simulink model "kinematic_on_real_system"  (R2016b)
settings: Solver=FixedStepAuto  StartTime=0.0  StopTime=100  FixedStep=0.04  RelTol=1e-3  EnableMultiTasking=on
values from neighbouring files (symbols this model uses):
  Cx = [0 0 1 0 0 0;0 0 0 1 0 0;0 0 0 0 1 0; 0 0 0 0 0 1]    [lqgfin.m]
  Cy = [1 0 0 0 0 0;0 1 0 0 0 0]    [lqgfin.m]
  l = 0.21    [lqgfin.m]
  ly = 0.1    [lqgfin.m]
  r = 0.13/2    (= 0.065)    [lqgfin.m]
  u_51 = [[-5:0.2:-3],[-2.9:0.1:2.9],[3:0.2:5]]    [lqgfin.m]
  vol_l = [-[10.3,9.95,9.86,9.8,9.74,9.65,9.53,9.42,9.3,9.15,8.98,8.86,     8.75,8.64,8.53,8.39,8.25,8.05,7.9,7.6,7.4,7.1,6.88,6.48,6.1,5.7,     5.2,4.7,4.13,3.45,2.7,1.75,0.21,0.165,0.12,0.088,0.06,0.036,0.017,     0.005],[0,0.005,0.017,0.035,0.061,0.092,0.122,0.160,0.960,1.7,2.6,     3.25,4,4.6,5.1,5.6,6,6.44,6.8,7.1,7.4,7.65,7.8,8,8.11,8.25,8.4,     8.55,8.68,8.82,8.95,9.15,9.29,9.44,9.56,9.67,9.75,9.82, ...(+23 chars)    [lqgfin.m]
  vol_r = [-[10.31,9.98,9.88,9.8,9.72,9.62,9.5,9.37,9.22,9.05,8.87,8.73,     8.62,8.49,8.35,8.19,8.01,7.84,7.63,7.41,7.16,6.76,6.43,6.09,5.68,     5.22,4.74,4.16,3.56,2.92,2.15,0.42,0.35,0.032,0.027,0.023,0.019,     0.013,0.0068,0.00156],[0,0.0013,0.0018,0.006,0.012,0.018,0.026,     0.032,0.109,1.16,2,2.67,3.35,4.05,4.61,5.12,5.59,6.00,6.35,6.69,     7.06,7.29,7.55,7.77,7.96,8.14,8.31,8.45,8.59,8.72,8.86,9. ...(+55 chars)    [lqgfin.m]
undefined symbols (not defined in the file or in its folder): An, Bn, Cn, codertarget, Dn, gcbh, K_lqi
libraries: simulink x9, arduinolib x4, Controllers x2, MinSegLibrary_M1V4 x2, DiffSteer_model x1
settings Model: SimulationMode=external  ExtModeTrigDuration=2  Creator=Hamza  LastModifiedBy=Hamza
settings OptimizationCC: MaxStackSize=64
settings DebuggingCC: ParameterTunabilityLossMsg=error
settings HardwareCC: ProdBitPerPointer=32  ProdBitPerSizeT=32  ProdBitPerPtrDiffT=32  ProdLargestAtomicInteger=Long  ProdLargestAtomicFloat=Double  ProdWordSize=32  ProdHWDeviceType=ARM Compatible->ARM Cortex
settings RTWCC: SystemTargetFile=ert.tlc  HardwareBoard=Arduino Due  TLCOptions=-aInlineSetEventsForThisBaseRateFcn=TLC_FALSE -aSuppressMultiTaskScheduler=TLC_FALSE -aRateBasedStepFcn=1  TemplateMakefile=ert_default_tmf  Description=Embedded Coder  GenerateReport=on  Toolchain=Arduino ARM  BuildConfiguration=Faster Runs  IncludeHyperlinkInReport=on  LaunchReport=on  GenerateTraceInfo=on  GenerateTraceReport=on  GenerateTraceReportSl=on  GenerateTraceReportSf=on  GenerateTraceReportEml=on
settings CodeAppCC: ForceParamTrailComments=on  IgnoreCustomStorageClasses=off  OperatorAnnotations=on  SimulinkDataObjDesc=on  SFDataObjDesc=on  MATLABFcnDesc=on  InsertBlockDesc=on  MATLABSourceComments=on
settings ERTTargetCC: SupportContinuousTime=on  SupportVariableSizeSignals=on  ExtMode=on  ExtModeMexArgs='127.0.0.1' 0 17725

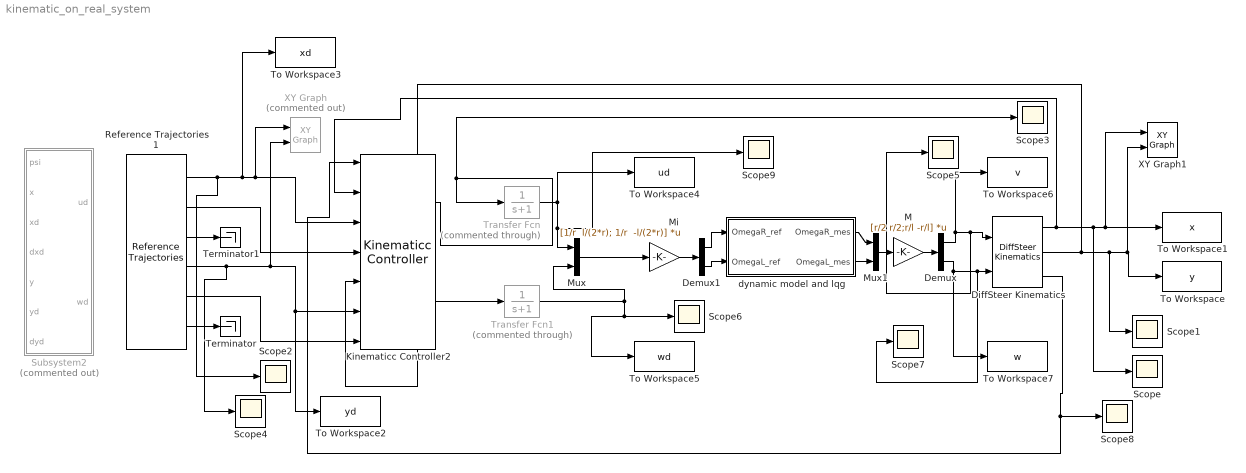
== system kinematic_on_real_system ==
  Demux : Demux  Outputs=2
  Demux1 : Demux  Outputs=2
  DiffSteer Kinematics : DiffSteer_model/DiffSteer Kinematics  x0=[0, 0, 0]  a=0.18  umax=1.3  wmax=12  dumax=5  dwmax=5
  Kinematicc Controller2 : Controllers/Kinematicc Controller  kx=1  ky=1  lx=0.25  ly=0.25  a=0
      link override 1//a: Gain=1/0.18
  M : Gain  Gain=[r/2 r/2;r/l -r/l]  Multiplication=Matrix(K*u)
  Mi : Gain  Gain="[1/r  l/(2*r); 1/r  -l/(2*r)]"  Multiplication=Matrix(K*u)
  Mux : Mux  Inputs=2
  Mux1 : Mux  Inputs=2
  Reference Trajectories1 : Controllers/Reference Trajectories  trajectory_type=1  wf=0.2  raio_ref_1=1.15  delta_raio=-0.1  t_delta_raio=100  xd=[2.5, 2.5]
      link override ganho: Gain=1
      link override zero2: Value=1
  Scope{,1..9} (10 alike) : Scope
  Subsystem2 : Subsystem  Commented=on
  Terminator : Terminator
  Terminator1 : Terminator
  To Workspace : ToWorkspace  VariableName=y  SampleTime=-1
  To Workspace1 : ToWorkspace  VariableName=x  SampleTime=-1
  To Workspace2 : ToWorkspace  VariableName=yd  SampleTime=-1
  To Workspace3 : ToWorkspace  VariableName=xd  SampleTime=-1
  To Workspace4 : ToWorkspace  VariableName=ud  SampleTime=-1
  To Workspace5 : ToWorkspace  VariableName=wd  SampleTime=-1
  To Workspace6 : ToWorkspace  VariableName=v  SampleTime=-1
  To Workspace7 : ToWorkspace  VariableName=w  SampleTime=-1
  Transfer Fcn : TransferFcn  Commented=through  Denominator=[1 1]
  Transfer Fcn1 : TransferFcn  Commented=through  Denominator=[1 1]
  XY Graph : simulink/Sinks/XY Graph  Commented=on  xmin=-2  xmax=50  ymin=-3  ymax=50  st=-1
  XY Graph1 : simulink/Sinks/XY Graph  xmin=-1.5  xmax=1.5  ymin=-1.5  ymax=1.5  st=-1
  dynamic model and lqg : Subsystem
  wires:
  Reference Trajectories1/1 -> Scope2/1, To Workspace3/1, Kinematicc Controller2/3, XY Graph/1
  Reference Trajectories1/2 -> Kinematicc Controller2/4
  Reference Trajectories1/4 -> Scope4/1, XY Graph/2, To Workspace2/1, Kinematicc Controller2/6
  Reference Trajectories1/5 -> Kinematicc Controller2/7
  DiffSteer Kinematics/1 -> Kinematicc Controller2/2, Scope/1, XY Graph1/1, To Workspace1/1
  DiffSteer Kinematics/2 -> Kinematicc Controller2/5, Scope1/1, XY Graph1/2, To Workspace/1
  DiffSteer Kinematics/3 -> Kinematicc Controller2/1, Scope8/1
  Kinematicc Controller2/2 -> Transfer Fcn1/1
  Demux/2 -> Scope7/1, DiffSteer Kinematics/2, To Workspace7/1
  Reference Trajectories1/3 -> Terminator1/1
  Reference Trajectories1/6 -> Terminator/1
  Mux1/1 -> M/1
  Mux/1 -> Mi/1
  M/1 -> Demux/1
  Mi/1 -> Demux1/1
  Demux1/1 -> dynamic model and lqg/1(OmegaR_ref)
  dynamic model and lqg/1(OmegaR_mes) -> Mux1/1
  dynamic model and lqg/2(OmegaL_mes) -> Mux1/2
  Demux/1 -> Scope5/1, DiffSteer Kinematics/1, To Workspace6/1
  Kinematicc Controller2/1 -> Transfer Fcn/1, Scope3/1
  Transfer Fcn/1 -> Scope9/1, Mux/1, To Workspace4/1
  Transfer Fcn1/1 -> To Workspace5/1, Scope6/1, Mux/2
  Demux1/2 -> dynamic model and lqg/2(OmegaL_ref)

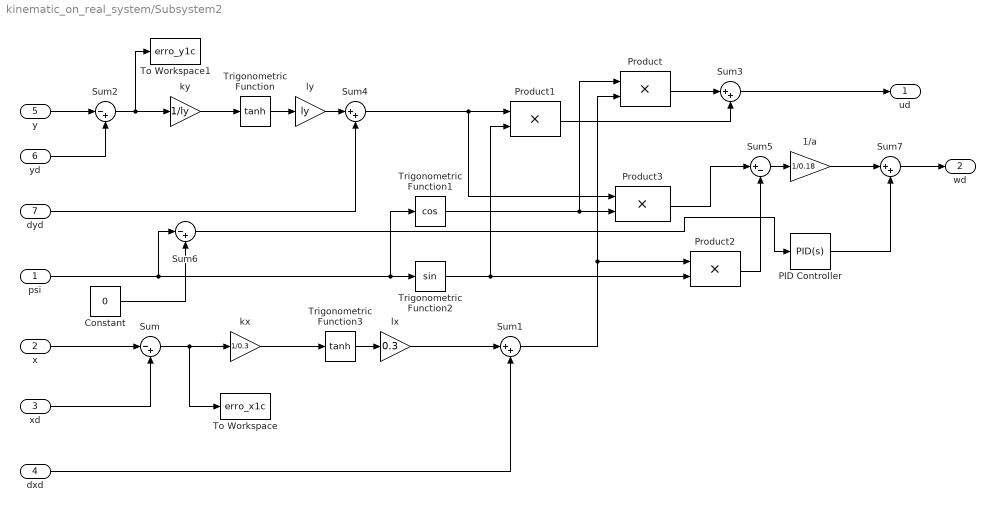
== system kinematic_on_real_system/Subsystem2 ==
  psi : Inport
  x : Inport  Port=2
  xd : Inport  Port=3
  dxd : Inport  Port=4
  y : Inport  Port=5
  yd : Inport  Port=6
  dyd : Inport  Port=7
  1/a : Gain  Gain=1/0.18  SaturateOnIntegerOverflow=on  OutDataTypeStr=Inherit: Same as input  ParamDataTypeStr=Inherit: Same as input
  Constant : Constant  Value=0
  PID Controller : simulink/Continuous/PID Controller  Controller=PID  TimeDomain=Continuous-time  SampleTime=-1  IntegratorMethod=Forward Euler  FilterMethod=Forward Euler  Form=Parallel  UseFilter=on  ControllerParametersSource=internal  P=1  I=0.01  D=0.5  N=100  InitialConditionSource=internal  InitialConditionForIntegrator=0  InitialConditionForFilter=0  ExternalReset=none  LimitOutput=off  UpperSaturationLimit=inf  LowerSaturationLimit=-inf  LinearizeAsGain=on  AntiWindupMode=none  Kb=1  TrackingMode=off  Kt=1  PParamMin=[]  PParamMax=[]  IParamMin=[]  IParamMax=[]  DParamMin=[]  DParamMax=[]  NParamMin=[]  NParamMax=[]  KbParamMin=[]  KbParamMax=[]  KtParamMin=[]  KtParamMax=[]  POutMin=[]  POutMax=[]  IOutMin=[]  IOutMax=[]  DOutMin=[]  DOutMax=[]  NOutMin=[]  NOutMax=[]  KbOutMin=[]  KbOutMax=[]  KtOutMin=[]  KtOutMax=[]  IntegratorOutMin=[]  IntegratorOutMax=[]  FilterOutMin=[]  FilterOutMax=[]  SumOutMin=[]  SumOutMax=[]  SumI1OutMin=[]  SumI1OutMax=[]  SumI2OutMin=[]  SumI2OutMax=[]  SumI3OutMin=[]  SumI3OutMax=[]  SumDOutMin=[]  SumDOutMax=[]  SaturationOutMin=[]  SaturationOutMax=[]  IntegratorContinuousStateAttributes=''  IntegratorStateMustResolveToSignalObject=off  IntegratorRTWStateStorageClass=Auto  FilterContinuousStateAttributes=''  FilterStateMustResolveToSignalObject=off  FilterRTWStateStorageClass=Auto  DifferentiatorICPrevScaledInput=0  DifferentiatorOutMin=[]  DifferentiatorOutMax=[]
  Product{,1..3} (4 alike) : Product  SaturateOnIntegerOverflow=on  OutDataTypeStr=Inherit: Same as first input
  Sum : Sum  Inputs=|-+  SaturateOnIntegerOverflow=on
  Sum{1,3..4,7} (4 alike) : Sum  Inputs=|++  SaturateOnIntegerOverflow=on
  Sum2 : Sum  Inputs=|-+  SaturateOnIntegerOverflow=on
  Sum5 : Sum  Inputs=|+-  SaturateOnIntegerOverflow=on
  Sum6 : Sum  Inputs=|-+  SaturateOnIntegerOverflow=on
  To Workspace : ToWorkspace  VariableName=erro_x1c  SampleTime=-1
  To Workspace1 : ToWorkspace  VariableName=erro_y1c  SampleTime=-1
  Trigonometric Function : Trigonometry  Operator=tanh
  Trigonometric Function1 : Trigonometry  Operator=cos
  Trigonometric Function2 : Trigonometry
  Trigonometric Function3 : Trigonometry  Operator=tanh
  kx : Gain  Gain=1/0.3  SaturateOnIntegerOverflow=on  OutDataTypeStr=Inherit: Same as input  ParamDataTypeStr=Inherit: Same as input
  ky : Gain  Gain=1/ly  SaturateOnIntegerOverflow=on  OutDataTypeStr=Inherit: Same as input  ParamDataTypeStr=Inherit: Same as input
  lx : Gain  Gain=0.3  SaturateOnIntegerOverflow=on  OutDataTypeStr=Inherit: Same as input  ParamDataTypeStr=Inherit: Same as input
  ly : Gain  Gain=ly  SaturateOnIntegerOverflow=on  OutDataTypeStr=Inherit: Same as input  ParamDataTypeStr=Inherit: Same as input
  ud : Outport
  wd : Outport  Port=2
  wires:
  Sum/1 -> kx/1, To Workspace/1
  y/1 -> Sum2/1
  Sum4/1 -> Product1/1, Product3/1
  Trigonometric Function2/1 -> Product2/2, Product1/2
  ky/1 -> Trigonometric Function/1
  kx/1 -> Trigonometric Function3/1
  Trigonometric Function1/1 -> Product3/2, Product/1
  yd/1 -> Sum2/2
  xd/1 -> Sum/2
  x/1 -> Sum/1
  psi/1 -> Sum6/1, Trigonometric Function2/1, Trigonometric Function1/1
  Sum1/1 -> Product2/1, Product/2
  Product1/1 -> Sum3/2
  Product3/1 -> Sum5/1
  Sum2/1 -> ky/1, To Workspace1/1
  Product/1 -> Sum3/1
  Product2/1 -> Sum5/2
  Sum3/1 -> ud/1
  ly/1 -> Sum4/1
  dxd/1 -> Sum1/2
  dyd/1 -> Sum4/2
  Trigonometric Function/1 -> ly/1
  lx/1 -> Sum1/1
  Trigonometric Function3/1 -> lx/1
  Sum7/1 -> wd/1
  Sum5/1 -> 1/a/1
  Sum6/1 -> PID Controller/1
  PID Controller/1 -> Sum7/2
  1/a/1 -> Sum7/1
  Constant/1 -> Sum6/2

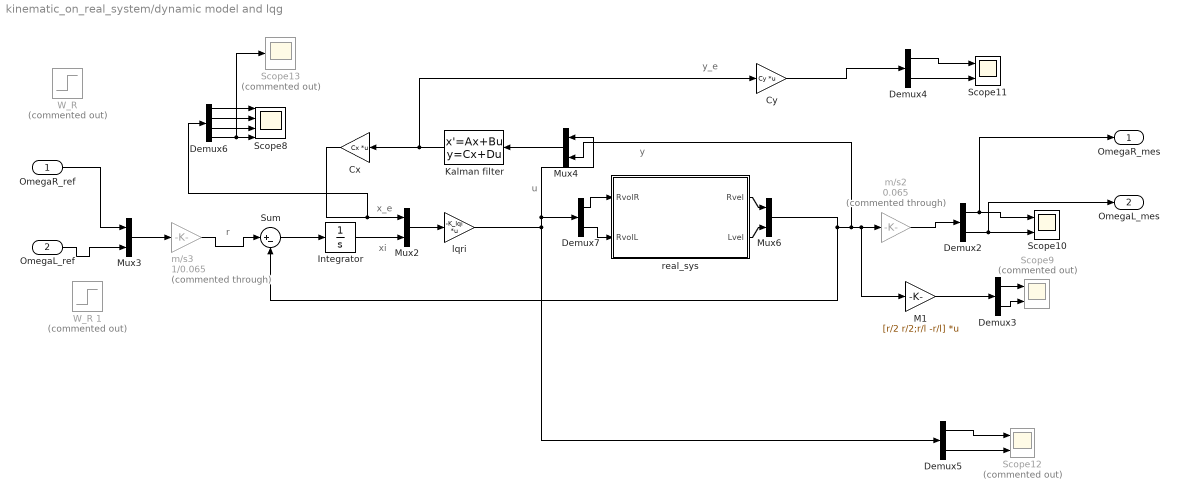
== system kinematic_on_real_system/dynamic model and lqg ==
  note: r
  note: y_e
  note: xi
  note: x_e
  note: u
  note: y
  OmegaR_ref : Inport
  OmegaL_ref : Inport  Port=2
  Cx : Gain  Gain=Cx  Multiplication=Matrix(K*u)
  Cy : Gain  Gain=Cy  Multiplication=Matrix(K*u)
  Demux{2..5,7} (5 alike) : Demux  Outputs=2
  Demux6 : Demux
  Integrator : Integrator
  Kalman filter : StateSpace  A=An  B=Bn  C=Cn  D=Dn  X0=0
  M1 : Gain  Gain=[r/2 r/2;r/l -r/l]  Multiplication=Matrix(K*u)
  Mux{2..4,6} (4 alike) : Mux  Inputs=2
  Scope10 : Scope  NumInputPorts=2
  Scope11 : Scope  NumInputPorts=2
  Scope12 : Scope  Commented=on  NumInputPorts=2
  Scope13 : Scope  Commented=on
  Scope8 : Scope  NumInputPorts=4
  Scope9 : Scope  Commented=on  NumInputPorts=2
  Sum : Sum  Inputs=|+-
  "W_R " : Step  Commented=on  After=10  SampleTime=0.02
  W_R 1 : Step  Commented=on  After=10  SampleTime=0.02
  lqri : Gain  Gain=-K_lqi  Multiplication=Matrix(K*u)
  m/s2 : Gain  Commented=through  Gain=0.065
  m/s3 : Gain  Commented=through  Gain=1/0.065
  "real_sys " : Subsystem
  OmegaR_mes : Outport
  OmegaL_mes : Outport  Port=2
  wires:
  OmegaR_ref/1 -> Mux3/1
  Demux5/1 -> Scope12/1
  Demux7/1 -> "real_sys "/1(RvolR)
  Demux5/2 -> Scope12/2
  "real_sys "/1(Rvel) -> Mux6/1
  Demux7/2 -> "real_sys "/2("RvolL ")
  lqri/1 -> Demux7/1, Mux4/1, Demux5/1
  "real_sys "/2(Lvel) -> Mux6/2
  Demux3/2 -> Scope9/2
  Cx/1 -> Demux6/1, Mux2/1
  M1/1 -> Demux3/1
  Demux6/1 -> Scope8/1
  Mux6/1 -> Sum/2, M1/1, m/s2/1, Mux4/2
  Demux6/2 -> Scope8/2
  Demux6/3 -> Scope8/3
  Demux6/4 -> Scope13/1, Scope8/4
  m/s2/1 -> Demux2/1
  Demux3/1 -> Scope9/1
  m/s3/1 -> Sum/1
  Cy/1 -> Demux4/1
  Sum/1 -> Integrator/1
  Integrator/1 -> Mux2/2
  Mux2/1 -> lqri/1
  Mux3/1 -> m/s3/1
  Demux2/2 -> OmegaL_mes/1, Scope10/2
  Kalman filter/1 -> Cy/1, Cx/1
  Demux4/1 -> Scope11/1
  Mux4/1 -> Kalman filter/1
  OmegaL_ref/1 -> Mux3/2
  Demux2/1 -> OmegaR_mes/1, Scope10/1
  Demux4/2 -> Scope11/2

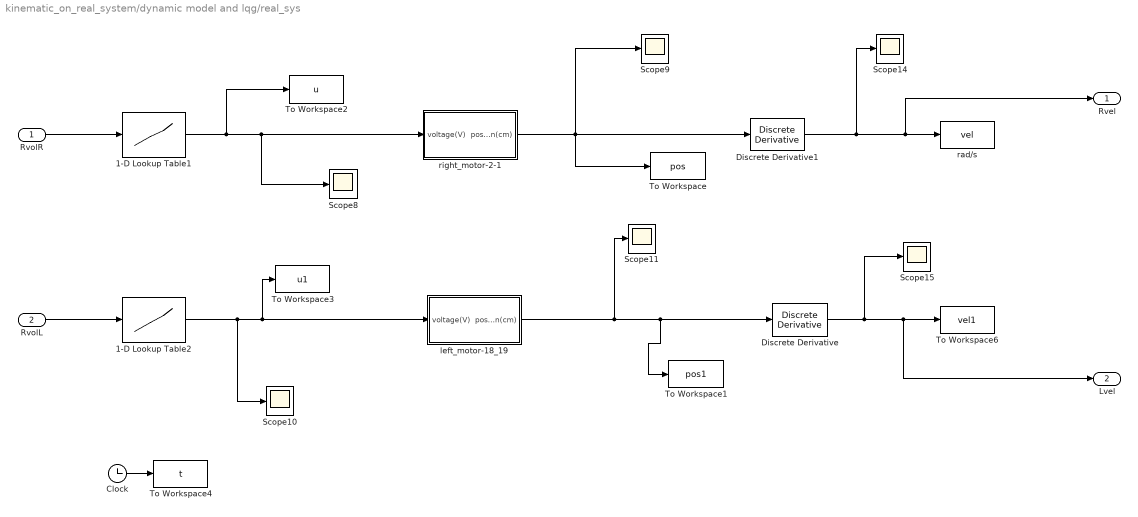
== system kinematic_on_real_system/dynamic model and lqg/real_sys  ==
  RvolR : Inport
  "RvolL " : Inport  Port=2
  1-D Lookup Table1 : Lookup_n-D  NumberOfTableDimensions=1  BreakpointsForDimension1=vol_r  Table=u_51  InternalRulePriority=Speed  RndMeth=Simplest  InputSameDT=on
  1-D Lookup Table2 : Lookup_n-D  NumberOfTableDimensions=1  BreakpointsForDimension1=vol_l  Table=u_51  InternalRulePriority=Speed  RndMeth=Simplest  InputSameDT=on
  Clock : Clock
  Discrete Derivative : simulink/Discrete/Discrete Derivative  gainval=1.0  ICPrevScaledInput=0.0  OutMin=[]  OutMax=[]  OutDataType=fixdt(1, 16)  OutScaling=2^-10  DoSatur=off
  Discrete Derivative1 : simulink/Discrete/Discrete Derivative  gainval=1.0  ICPrevScaledInput=0.0  OutMin=[]  OutMax=[]  OutDataType=fixdt(1, 16)  OutScaling=2^-10  DoSatur=off
  Scope{8..11,14..15} (6 alike) : Scope
  To Workspace : ToWorkspace  VariableName=pos  SampleTime=-1
      settings: Save2DSignal=2-D array (concatenate along first dimension)
  To Workspace1 : ToWorkspace  VariableName=pos1  SampleTime=-1
      settings: Save2DSignal=2-D array (concatenate along first dimension)
  To Workspace2 : ToWorkspace  VariableName=u  SampleTime=-1
      settings: Save2DSignal=2-D array (concatenate along first dimension)
  To Workspace3 : ToWorkspace  VariableName=u1  SampleTime=-1
      settings: Save2DSignal=2-D array (concatenate along first dimension)
  To Workspace4 : ToWorkspace  VariableName=t  SampleTime=-1
      settings: Save2DSignal=2-D array (concatenate along first dimension)
  To Workspace6 : ToWorkspace  VariableName=vel1  SampleTime=-1
      settings: Save2DSignal=2-D array (concatenate along first dimension)
  "left_motor-18_19 " : Subsystem
  rad/s : ToWorkspace  VariableName=vel  SampleTime=-1
      settings: Save2DSignal=2-D array (concatenate along first dimension)
  right_motor-2-1 : Subsystem
  Rvel : Outport
  Lvel : Outport  Port=2
  wires:
  1-D Lookup Table1/1 -> To Workspace2/1, Scope8/1, right_motor-2-1/1(voltage(V))
  1-D Lookup Table2/1 -> Scope10/1, "left_motor-18_19 "/1(voltage(V)), To Workspace3/1
  right_motor-2-1/1(position(cm)) -> To Workspace/1, Scope9/1, Discrete Derivative1/1
  RvolR/1 -> 1-D Lookup Table1/1
  "RvolL "/1 -> 1-D Lookup Table2/1
  Discrete Derivative1/1 -> Scope14/1, Rvel/1, rad/s/1
  Discrete Derivative/1 -> Scope15/1, Lvel/1, To Workspace6/1
  "left_motor-18_19 "/1(position(cm)) -> Discrete Derivative/1, To Workspace1/1, Scope11/1
  Clock/1 -> To Workspace4/1

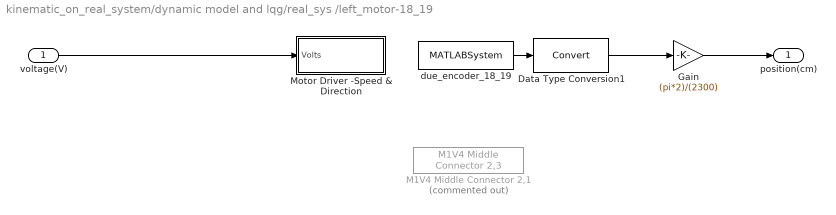
== system kinematic_on_real_system/dynamic model and lqg/real_sys /left_motor-18_19  ==
  voltage(V) : Inport
  Data Type Conversion1 : DataTypeConversion
  Gain : Gain  Gain=(pi*2)/(2300)
  M1V4 Middle Connector 2,1 : MinSegLibrary_M1V4/M1V4 Middle Connector 2,3  Commented=on  Encoder=1  PinA=18  PinB=19  PWMFSelect=1  PWMTimer=-1  SampleTime=-1
  Motor Driver -Speed & Direction : Subsystem  AncestorBlock=RASPlib/Motor Driver -Speed & Direction  mask(Motor Driver){Vsupply=5, PWMPin=5, DigitalPin=4}
      mask prompts: Vsupply "Driver Voltage"; PWMPin "PWM Pin"; DigitalPin "Digital Pin"
      mask help:
      | Use a single PWM and a single Digtial out to control the magnitude and direction of a motor
      |
      | Specify driver supply voltage (3.25 for USB with SN754410)
      mask Display:
      | port_label('input',1,'Volts')
      | text(15,5,['Vsupply=' num2str(Vsupply)])
  "due_encoder_18_19 " : MATLABSystem  System=Encoder_arduino_Due_18_19  Encoder=1  PinA=18  PinB=19  PWMFSelect=1  PWMTimer=-1  SampleTime=-1
      mask Type: Encoder_arduino_Due_18_19
      mask Display:
      | disp('soEncoder');
      | port_label('output',1,'y');
  position(cm) : Outport
  wires:
  voltage(V)/1 -> Motor Driver -Speed & Direction/1(Volts)
  "due_encoder_18_19 "/1 -> Data Type Conversion1/1
  Data Type Conversion1/1 -> Gain/1
  Gain/1 -> position(cm)/1

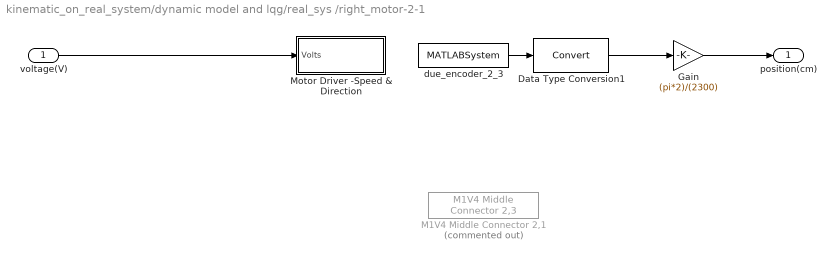
== system kinematic_on_real_system/dynamic model and lqg/real_sys /right_motor-2-1 ==
  voltage(V) : Inport
  Data Type Conversion1 : DataTypeConversion
  Gain : Gain  Gain=(pi*2)/(2300)
  M1V4 Middle Connector 2,1 : MinSegLibrary_M1V4/M1V4 Middle Connector 2,3  Commented=on  Encoder=0  PinA=2  PinB=3  PWMFSelect=1  PWMTimer=-1  SampleTime=-1
  Motor Driver -Speed & Direction : Subsystem  AncestorBlock=RASPlib/Motor Driver -Speed & Direction  mask(Motor Driver){Vsupply=5, PWMPin=5, DigitalPin=4}
      mask prompts: Vsupply "Driver Voltage"; PWMPin "PWM Pin"; DigitalPin "Digital Pin"
      mask help:
      | Use a single PWM and a single Digtial out to control the magnitude and direction of a motor
      |
      | Specify driver supply voltage (3.25 for USB with SN754410)
      mask Display:
      | port_label('input',1,'Volts')
      | text(15,5,['Vsupply=' num2str(Vsupply)])
  due_encoder_2_3 : MATLABSystem  System=Encoder_arduino_Due_2_3  Encoder=0  PinA=2  PinB=3  PWMFSelect=1  PWMTimer=-1  SampleTime=-1
      mask Type: Encoder_arduino_Due_2_3
      mask Display:
      | disp('soEncoder');
      | port_label('output',1,'y');
  position(cm) : Outport
  wires:
  Gain/1 -> position(cm)/1
  Data Type Conversion1/1 -> Gain/1
  due_encoder_2_3/1 -> Data Type Conversion1/1
  voltage(V)/1 -> Motor Driver -Speed & Direction/1(Volts)

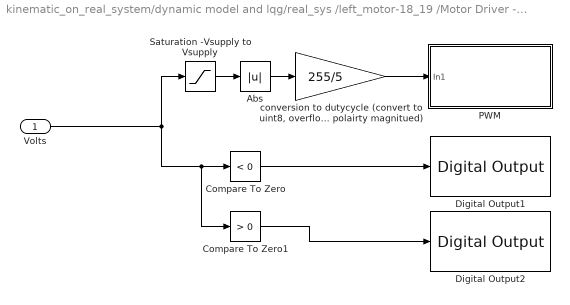
== system kinematic_on_real_system/dynamic model and lqg/real_sys /left_motor-18_19 /Motor Driver -Speed & Direction ==
  Volts : Inport
  Abs : Abs
  Compare To Zero : simulink/Logic and Bit Operations/Compare To Zero  relop=<  OutDataTypeStr=boolean
  Compare To Zero1 : simulink/Logic and Bit Operations/Compare To Zero  relop=>  OutDataTypeStr=boolean
  Digital Output1 : arduinolib/Digital Output  pinNumber=8  blockPlatform=arduino
  Digital Output2 : arduinolib/Digital Output  pinNumber=7  blockPlatform=arduino
  PWM : Subsystem  AncestorBlock=arduinolib/PWM  InitFcn=codertarget.arduinobase.blocks.arduinoBlockInitFcnCallback(gcbh);  mask(Arduino PWM){pinNumber=9, blockPlatform=arduino}
      mask prompts: pinNumber "Pin number:"; blockPlatform "Block platform:"
      mask help:
      | Generate square waveform on the specified analog output pin. The block input controls the duty cycle of the square waveform. An input value of 0 produces a 0 percent duty cycle, and an input value of 255 produces a 100 percent duty cycle. The frequency of the waveform is constant at approximately 490 Hz.
      |
      | Enter the number of the analog output pin. Do not assign the same pin number to multiple blocks within a model.
      mask init:
      | codertarget.arduinobase.blocks.registerPWMBlock(gcbh);
      | codertarget.arduinobase.blocks.arduinoAnalogOutputCallback('MaskInitialization');
      mask Help: eval('codertarget.internal.helpView(''arduinoert'', ''arduinolibarduinopwm'')')
      mask DialogControl Control2 Prompt: View pin map
      mask DialogControl Control2 Callback:
      | file = [codertarget.arduinobase.internal.getBaseSpPkgRootDir filesep 'blocks' filesep 'mex' filesep 'arduinoPinMapping.html'];
      | web(file)
      mask Display:
      | pic=imread('analogoutpwm.png');image(pic,[0.32 0.25 0.35 0.55]);text(0.5, 0.15, 'Pin 9', 'horizontalAlignment', 'center');
      | color('blue');
      | text(0.55, 0.87, 'ARDUINO', 'horizontalAlignment', 'left');
      | color('black');
  Saturation -Vsupply to Vsupply : Saturate  UpperLimit=5  LowerLimit=-5  OutDataTypeStr=single
  "conversion to dutycycle (convert to uint8, overflow will provide reverse polairty magnitued)" : Gain  Gain=255/5  OutDataTypeStr=uint8
  wires:
  Volts/1 -> Compare To Zero1/1, Compare To Zero/1, Saturation -Vsupply to Vsupply/1
  Saturation -Vsupply to Vsupply/1 -> Abs/1
  "conversion to dutycycle (convert to uint8, overflow will provide reverse polairty magnitued)"/1 -> PWM/1(In1)
  Compare To Zero/1 -> Digital Output1/1
  Compare To Zero1/1 -> Digital Output2/1
  Abs/1 -> "conversion to dutycycle (convert to uint8, overflow will provide reverse polairty magnitued)"/1

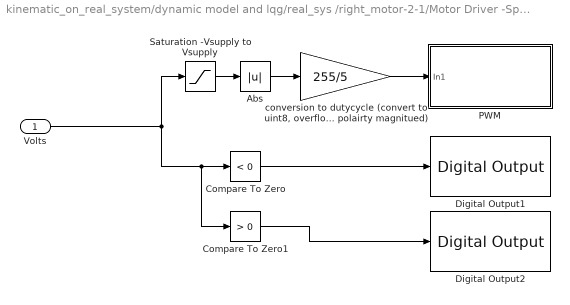
== system kinematic_on_real_system/dynamic model and lqg/real_sys /right_motor-2-1/Motor Driver -Speed & Direction ==
  Volts : Inport
  Abs : Abs
  Compare To Zero : simulink/Logic and Bit Operations/Compare To Zero  relop=<  OutDataTypeStr=boolean
  Compare To Zero1 : simulink/Logic and Bit Operations/Compare To Zero  relop=>  OutDataTypeStr=boolean
  Digital Output1 : arduinolib/Digital Output  pinNumber=6  blockPlatform=arduino
  Digital Output2 : arduinolib/Digital Output  pinNumber=5  blockPlatform=arduino
  PWM : Subsystem  AncestorBlock=arduinolib/PWM  InitFcn=codertarget.arduinobase.blocks.arduinoBlockInitFcnCallback(gcbh);  mask(Arduino PWM){pinNumber=4, blockPlatform=arduino}
      mask prompts: pinNumber "Pin number:"; blockPlatform "Block platform:"
      mask help:
      | Generate square waveform on the specified analog output pin. The block input controls the duty cycle of the square waveform. An input value of 0 produces a 0 percent duty cycle, and an input value of 255 produces a 100 percent duty cycle. The frequency of the waveform is constant at approximately 490 Hz.
      |
      | Enter the number of the analog output pin. Do not assign the same pin number to multiple blocks within a model.
      mask init:
      | codertarget.arduinobase.blocks.registerPWMBlock(gcbh);
      | codertarget.arduinobase.blocks.arduinoAnalogOutputCallback('MaskInitialization');
      mask Help: eval('codertarget.internal.helpView(''arduinoert'', ''arduinolibarduinopwm'')')
      mask DialogControl Control2 Prompt: View pin map
      mask DialogControl Control2 Callback:
      | file = [codertarget.arduinobase.internal.getBaseSpPkgRootDir filesep 'blocks' filesep 'mex' filesep 'arduinoPinMapping.html'];
      | web(file)
      mask Display:
      | pic=imread('analogoutpwm.png');image(pic,[0.32 0.25 0.35 0.55]);text(0.5, 0.15, 'Pin 4', 'horizontalAlignment', 'center');
      | color('blue');
      | text(0.55, 0.87, 'ARDUINO', 'horizontalAlignment', 'left');
      | color('black');
  Saturation -Vsupply to Vsupply : Saturate  UpperLimit=5  LowerLimit=-5  OutDataTypeStr=single
  "conversion to dutycycle (convert to uint8, overflow will provide reverse polairty magnitued)" : Gain  Gain=255/5  OutDataTypeStr=uint8
  wires:
  Abs/1 -> "conversion to dutycycle (convert to uint8, overflow will provide reverse polairty magnitued)"/1
  Compare To Zero1/1 -> Digital Output2/1
  Compare To Zero/1 -> Digital Output1/1
  "conversion to dutycycle (convert to uint8, overflow will provide reverse polairty magnitued)"/1 -> PWM/1(In1)
  Saturation -Vsupply to Vsupply/1 -> Abs/1
  Volts/1 -> Saturation -Vsupply to Vsupply/1, Compare To Zero/1, Compare To Zero1/1

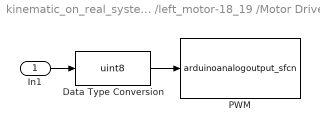
== system kinematic_on_real_system/dynamic model and lqg/real_sys /left_motor-18_19 /Motor Driver -Speed & Direction/PWM ==
  In1 : Inport
  Data Type Conversion : DataTypeConversion  OutDataTypeStr=uint8  SaturateOnIntegerOverflow=on
  PWM : S-Function  FunctionName=arduinoanalogoutput_sfcn  Parameters=pinNumber  SFunctionDeploymentMode=off  EnableBusSupport=off  mask(Arduino Analog Output Core){pinNumber=9}
      mask prompts: pinNumber "Pin number:"
      mask Display: pic=imread('analogoutpwm.png');image(pic,[0.32 0.25 0.35 0.55]);
  wires:
  In1/1 -> Data Type Conversion/1
  Data Type Conversion/1 -> PWM/1

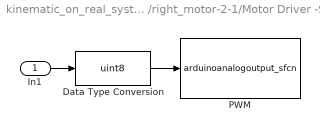
== system kinematic_on_real_system/dynamic model and lqg/real_sys /right_motor-2-1/Motor Driver -Speed & Direction/PWM ==
  In1 : Inport
  Data Type Conversion : DataTypeConversion  OutDataTypeStr=uint8  SaturateOnIntegerOverflow=on
  PWM : S-Function  FunctionName=arduinoanalogoutput_sfcn  Parameters=pinNumber  SFunctionDeploymentMode=off  EnableBusSupport=off  mask(Arduino Analog Output Core){pinNumber=4}
      mask prompts: pinNumber "Pin number:"
      mask Display: pic=imread('analogoutpwm.png');image(pic,[0.32 0.25 0.35 0.55]);
  wires:
  Data Type Conversion/1 -> PWM/1
  In1/1 -> Data Type Conversion/1
